simulink model "Diagrama_entrada_triangular_tempo_continuo"  (R2022b)
settings: Solver=VariableStepAuto  StartTime=0.0  StopTime=100  RelTol=1e-3
values from neighbouring files (symbols this model uses):
  betha = n    (= 7)    [Q1.m]    (also in Q2_raizes.m = 2.85714285714)
  betha_e = 20/n    (= 2.85714285714)    [Q2_raizes.m]
  g = 9.8    [Q2_raizes.m]
  Jm = n    (= 7)    [Q2_raizes.m]
  Kb = 0.1*n    (= 0.7)    [Q2_raizes.m]
  Ki = 20/n    (= 2.85714285714)    [Q2_raizes.m]
  La = 0.1*n    (= 0.7)    [Q2_raizes.m]
  m = sqrt(1/n)    [Q2_raizes.m]
  n = 7    [Q1.m]    (also in Q2_raizes.m)
  Ra = 20/n    (= 2.85714285714)    [Q2_raizes.m]
libraries: simulink x1
settings Model: Creator=kaiqu  LastModifiedBy=kaiqu

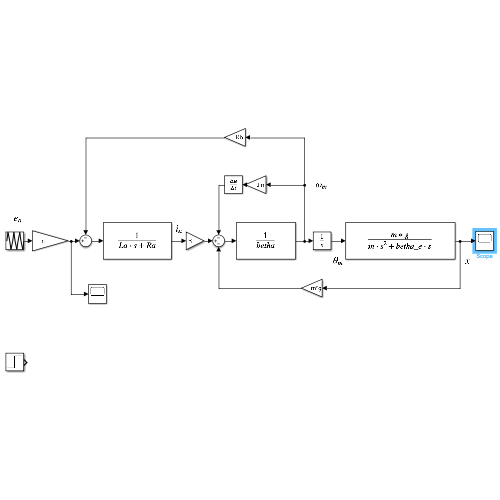
[thumbnail: Simulink's stored preview of the top-level diagram]
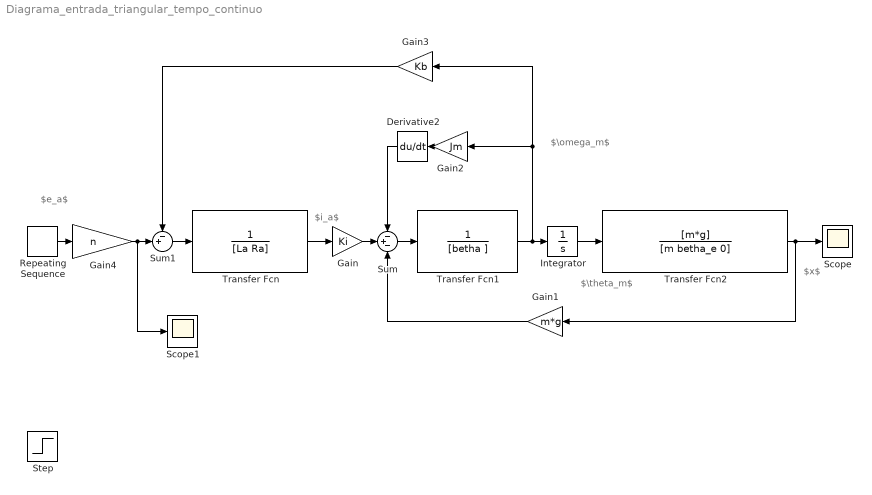
== system Diagrama_entrada_triangular_tempo_continuo ==
  note: $\omega_m$
  note: $\theta_m$
  note: $x$
  note: $i_a$
  note: $e_a$
  Derivative2 : Derivative
  Gain : Gain  Gain=Ki
  Gain1 : Gain  Gain=m*g
  Gain2 : Gain  Gain=Jm
  Gain3 : Gain  Gain=Kb
  Gain4 : Gain  Gain=n
  Integrator : Integrator
  Repeating Sequence : simulink/Sources/Repeating Sequence  rep_seq_t=[0 1 2 3 4]  rep_seq_y=[0 0.01 0 -0.01 0]
  Scope : Scope
  Scope1 : Scope
  Step : Step  SampleTime=0
  Sum : Sum  Inputs=-+-
  Sum1 : Sum  Inputs=-+|
  Transfer Fcn : TransferFcn  Denominator=[La Ra]
  Transfer Fcn1 : TransferFcn  Denominator=[betha ]
  Transfer Fcn2 : TransferFcn  Numerator=[m*g]  Denominator=[m betha_e 0]
  wires:
  Transfer Fcn/1 -> Gain/1
  Gain/1 -> Sum/2
  Sum/1 -> Transfer Fcn1/1
  Transfer Fcn2/1 -> Gain1/1, Scope/1
  Gain1/1 -> Sum/3
  Transfer Fcn1/1 -> Integrator/1, Gain2/1, Gain3/1
  Gain2/1 -> Derivative2/1
  Derivative2/1 -> Sum/1
  Sum1/1 -> Transfer Fcn/1
  Gain3/1 -> Sum1/1
  Integrator/1 -> Transfer Fcn2/1
  Repeating Sequence/1 -> Gain4/1
  Gain4/1 -> Scope1/1, Sum1/2
